simulink model "DSBSC_MODULATOR_DEMODULATOR"  (R2023a)
settings: Solver=VariableStepAuto  StartTime=0.0  StopTime=1  RelTol=1e-3
libraries: dspfdesign x1
settings Model: Creator=Pedro  LastModifiedBy=Pedro

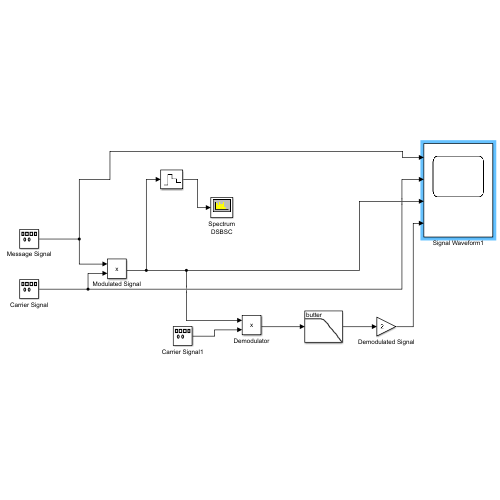
[thumbnail: Simulink's stored preview of the top-level diagram]
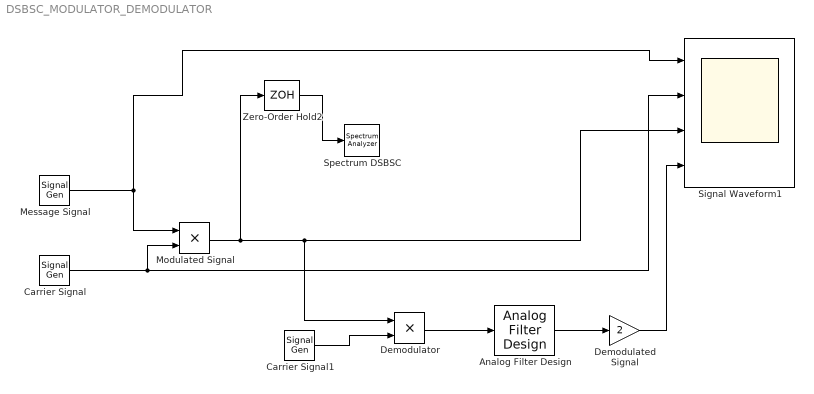
== system DSBSC_MODULATOR_DEMODULATOR ==
  Analog Filter Design : dspfdesign/Analog Filter Design  method=Butterworth  filttype=Lowpass  N=4  Wlo=2*pi*40  Whi=80  Rp=2  Rs=40
  Carrier Signal : SignalGenerator  Frequency=110
  Carrier Signal1 : SignalGenerator  Frequency=110
  Demodulated Signal : Gain  Gain=2
  Demodulator : Product
  Message Signal : SignalGenerator  Amplitude=1.5  Frequency=20
  Modulated Signal : Product
  Signal Waveform1 : Scope  NumInputPorts=4
  Spectrum DSBSC : SpectrumAnalyzer  WindowPosition=[1.000000,41.000000,1280.000000,657.000000,]  ScopeFrameLocation=window  Method=Welch  PlotAsTwoSidedSpectrum=off  Span=100  CenterFrequency=250  SpectrumUnits=Watts  YLimits=[-0.03496899,0.31472088]  ColorLimits=[-80 20]  SelectedToolstripTab=spectrumAnalyzerToolstrip.estimationTab
  Zero-Order Hold2 : ZeroOrderHold  SampleTime=0.0001
  wires:
  Message Signal/1 -> Signal Waveform1/1, Modulated Signal/1
  Carrier Signal/1 -> Signal Waveform1/2, Modulated Signal/2
  Modulated Signal/1 -> Signal Waveform1/3, Demodulator/1, Zero-Order Hold2/1
  Carrier Signal1/1 -> Demodulator/2
  Demodulator/1 -> Analog Filter Design/1
  Zero-Order Hold2/1 -> Spectrum DSBSC/1
  Analog Filter Design/1 -> Demodulated Signal/1
  Demodulated Signal/1 -> Signal Waveform1/4
